simulink model "RaibertControlV13"  (R2022a)
settings: Solver=ode23t  StartTime=0.0  StopTime=10  FixedStep=1/1000  MaxStep=0.001  RelTol=1e-3  AbsTol=1e-3  EnableMultiTasking=on
values from neighbouring files (symbols this model uses):
  dphi_d_14 = 0.0    (= 0)    [initialization.m]
  dphi_d_23 = 0.0    (= 0)    [initialization.m]
  dphi_des = DesiredImpedenceValues(4)    [Controller.m]    (also in initialization.m = 0)
  dr_d_14 = 0.0    (= 0)    [initialization.m]
  dr_d_23 = 0.0    (= 0)    [initialization.m]
  dr_des = DesiredImpedenceValues(3)    [Controller.m]    (also in initialization.m = 0)
  Fpush_d_14 = 300    [initialization.m]
  Fpush_d_23 = 300    [initialization.m]
  GAIN_dx_d_14 = 0.05    [initialization.m]
  GAIN_dx_d_23 = 0.05    [initialization.m]
  join_legs = -1    [initialization.m]
  Kd_phi_d_14 = 10    [initialization.m]
  Kd_phi_d_23 = 10    [initialization.m]
  Kd_r_d_14 = Kp_r_d_14*0.1    (= 60)    [initialization.m]
  Kd_r_d_23 = Kp_r_d_23*0.1    (= 50)    [initialization.m]
  Kdphi_des = DesiredImpedenceValues(8)    [Controller.m]    (also in initialization.m = 5)
  Kdr_des = DesiredImpedenceValues(6)    [Controller.m]    (also in initialization.m = 700)
  Kp_phi_d_14 = 200    [initialization.m]
  Kp_phi_d_23 = 200    [initialization.m]
  Kp_r_d_14 = 600    [initialization.m]
  Kp_r_d_23 = 500    [initialization.m]
  Kpphi_des = DesiredImpedenceValues(7)    [Controller.m]    (also in initialization.m = 50)
  Kpr_des = DesiredImpedenceValues(5)    [Controller.m]    (also in initialization.m = 700)
  phi_d_14 = 0    [initialization.m]
  phi_d_23 = 0    [initialization.m]
  phi_des = DesiredImpedenceValues(2)    [Controller.m]    (also in initialization.m = 0)
  r_d_14 = 0.38    [initialization.m]
  r_d_23 = 0.38    [initialization.m]
  r_des = DesiredImpedenceValues(1)    [Controller.m]    (also in initialization.m = 0.4)
  rthrust_d_14 = 0.3    [initialization.m]
  rthrust_d_23 = 0.3    [initialization.m]
undefined symbols (not defined in the file or in its folder): Carrier, N, Ring, T, X, Y, Z
libraries: sm_lib x160, nesl_utility x25, Multibody_Parts_Lib x4, fl_lib x4
(part 1 of 8)
settings Model: Creator=user  LastModifiedBy=user
settings SolverCC: AutoScaleAbsTol=off  ZeroCrossAlgorithm=Adaptive  AutoInsertRateTranBlk=on  MaxZcPerStep=1
settings DataIOCC: LimitDataPoints=on  MaxDataPoints=10000
settings OptimizationCC: LifeSpan=inf
settings DebuggingCC: UnconnectedInputMsg=warning  UnconnectedOutputMsg=warning  UnconnectedLineMsg=warning  AllowSymbolicDim=off  SFUnexpectedBacktrackingDiag=warning  SFNoUnconditionalDefaultTransitionDiag=warning  SFExecutionAtInitializationDiag=none  SFMachineParentedDataDiag=warning  ArithmeticOperatorsInVariantConditions=warning
settings SFSimCC: SimUseLocalCustomCode=off  CustomCodeUndefinedFunction=UseInterfaceOnly
settings RTWCC: RTWUseLocalCustomCode=off  DLArmComputeVersion=19.05
settings CodeAppCC: StateflowObjectComments=on
settings GRTTargetCC: TargetLangStandard=C89/C90 (ANSI)
settings ConfigComp: CovMetricSettings=dw  CovSaveCumulativeToWorkspaceVar=on  CovSaveSingleToWorkspaceVar=on  CovExternalEMLEnable=off  CovSFcnEnable=off
settings SimscapeCC: SimscapeLogType=all  SimscapeLogSimulationStatistics=on  SimscapeLogDataHistory=10000
settings ExplorerConfigSet: InternalSimMechanicsExplorerSettings="<ExplorerConfiguration><canonicalview>planar_xy</canonicalview><AnimationSetting><BasePlaybackSpeed>1.0</BasePlaybackSpeed><PlaybackSpeedFactor>1.0</PlaybackSpeedFactor></AnimationSetting><TilePanel><TileInfo><Tiles Columns=\"1\" Count=\"1\" Rows=\"1\"><Column Weight=\"1\"/><Row Weight=\"1\"/><Tile Height=\"1\" Width=\"1\" X=\"0\" Y=\"0\"/></Tiles></TileInfo><SceneInfo><SceneViewer><BGColor><R>0.60000002384185791</R><G>0.60000002384185791</G><B>0.60000002384185791</B></BGColor><Camera><DoPerspective>off</DoPerspective><Position><X>-1.06238065184303165</X><Y>0.28591497324730003</Y><Z>-0.103858662281123768</Z></Position><Center><X>0.999999918886055106</X><Y>0.28591497324730003</Y><Z>-0.103858662281123768</Z></Center><Up><X>-0</X><Y>1</Y><Z>0</Z></Up><ViewLimDist>1</ViewLimDist><YLim>0.282634040177624779</YLim><XLim>0.661062811059710653</XLim></Camera></SceneViewer></SceneInfo></TilePanel><MechEditorPanel><Cameras/><GfxPanelCameraMap/><VideoCreator><PlaybackSpeedRatio>1.0</PlaybackSpeedRatio><FrameRate>30</FrameRate><VideoFormat>Motion JPEG AVI</VideoFormat><FrameSize>auto</FrameSize></VideoCreator></MechEditorPanel></ExplorerConfiguration>"

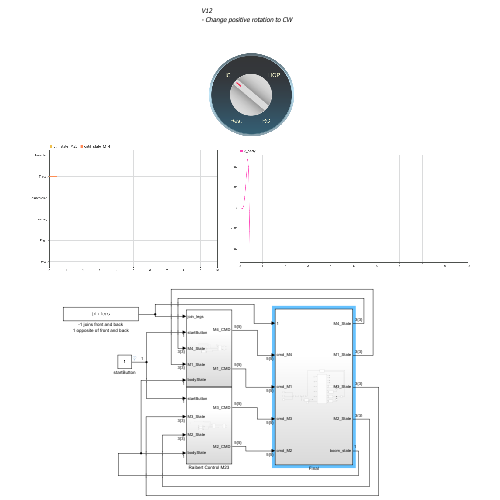
[thumbnail: Simulink's stored preview of the top-level diagram]
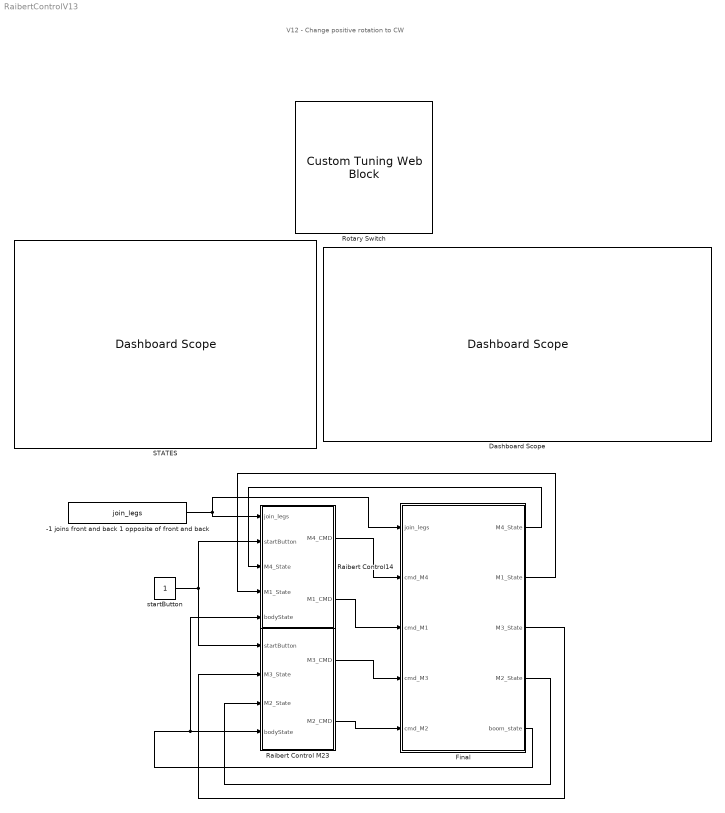
== system RaibertControlV13 ==
  note: V12
      | - Change positive rotation to CW
  -1 joins front and back 1 opposite of front and back : Constant  Value=join_legs
  Dashboard Scope : DashboardScope
  Final : Subsystem
  Raibert Control M23 : Subsystem
  Raibert Control14 : Subsystem
  Rotary Switch : CustomTuningWebBlock  LabelPosition=Hide  ShowInitialText=on  Configuration="{\"components\":[{\"name\":\"RotarySwitchComponent\",\"settings\":{\"arcAngle\":300,\"arcAngleOffset\":120,\"handle\":{\"size\":[150,150],\"src\":\"data:image\\/svg+xml;base64,PHN2ZyBpZD0iTGF5ZXJfMSIgZGF0YS1uYW1lPSJMYXllciAxIiB4bWxucz0iaHR0cDovL3d3dy53My5vcmcvMjAwMC9zdmciIHhtbG5zOnhsaW5rPSJodHRwOi8vd3d3LnczLm9yZy8xOTk5L3hsaW5rIiB2aWV3Qm94PSIwIDAgMTIxIDEyMSI+PGRlZnM+PHN0eWxlPi5jbHMtMXtmaWxsOnVybCgjbGluZWFyLWdyYWRpZW50KTt9LmNscy0yLC5jbHMtM3tmaWxsOiNkMWQxZDE7fS5jbHMtM3tzdHJva2U6I2I3YjdiNztzdHJva2UtbWl0ZXJsaW1pdDoxMDtzdHJva2Utd2lkdGg6MC4yNXB4O30uY2xzLTR7ZmlsbDojZjMwMDAwO30uY2xzLTV7ZmlsbDojZjIxNzY3O308L3N0eWxlPjxsaW5lYXJHcmFkaWVudCBpZD0ibGluZWFyLWdyYWRpZW50IiB4MT0iNjAuNSIgeTE9IjEyMC41IiB4Mj0iNjAuNSIgeTI9IjAuNSIgZ3JhZGllbnRVbml0cz0idXNlclNwYWNlT25Vc2UiPjxzdG9wIG9mZnNldD0iMCIgc3RvcC1jb2xvcj0iI2QxZDFkMSIvPjxzdG9wIG9mZnNldD0iMC4xIiBzdG9wLWNvbG9yPSIjY2VjZWNlIi8+PHN0b3Agb2Zmc2V0PSIwLjE5IiBzdG9wLWNvbG9yPSIjYzNjM2MzIi8+PHN0b3Agb2Zmc2V0PSIwLjI4IiBzdG9wLWNvbG9yPSIjYjFiMWIxIi8+PHN0b3Agb2Zmc2V0PSIwLjM2IiBzdG9wLWNvbG9yPSIjOTg5ODk4Ii8+PHN0b3Agb2Zmc2V0PSIwLjQ0IiBzdG9wLWNvbG9yPSIjNzg3ODc4Ii8+PHN0b3Agb2Zmc2V0PSIwLjQ2IiBzdG9wLWNvbG9yPSIjNmI2YjZiIi8+PHN0b3Agb2Zmc2V0PSIwLjU0IiBzdG9wLWNvbG9yPSIjNmI2YjZiIi8+PHN0b3Agb2Zmc2V0PSIwLjU2IiBzdG9wLWNvbG9yPSIjNzY3Njc2Ii8+PHN0b3Agb2Zmc2V0PSIwLjY0IiBzdG9wLWNvbG9yPSIjOTc5Nzk3Ii8+PHN0b3Agb2Zmc2V0PSIwLjcyIiBzdG9wLWNvbG9yPSIjYjBiMGIwIi8+PHN0b3Agb2Zmc2V0PSIwLjgxIiBzdG9wLWNvbG9yPSIjYzNjM2MzIi8+PHN0b3Agb2Zmc2V0PSIwLjkiIHN0b3AtY29sb3I9IiNjZGNkY2QiLz48c3RvcCBvZmZzZXQ9IjEiIHN0b3AtY29sb3I9IiNkMWQxZDEiLz48L2xpbmVhckdyYWRpZW50PjwvZGVmcz48Y2lyY2xlIGNsYXNzPSJjbHMtMSIgY3g9IjYwLjUiIGN5PSI2MC41IiByPSI2MCIvPjxwYXRoIGNsYXNzPSJjbHMtMiIgZD0iTTYwLjUsMUE1OS41LDU5LjUsMCwxLDEsMSw2MC41LDU5LjU3LDU5LjU3LDAsMCwxLDYwLjUsMW0wLTFBNjAuNSw2MC41LDAsMSwwLDEyMSw2MC41LDYwLjUsNjAuNSwwLDAsMCw2MC41LDBaIi8+PHJlY3QgY2xhc3M9ImNscy0zIiB4PSIwLjUiIHk9IjUxLjUiIHdpZHRoPSIxMjAiIGhlaWdodD0iMTgiIHJ4PSIzLjA0Ii8+PHJlY3QgY2xhc3M9ImNscy00IiB4PSI1Ljc1IiB5PSI1OC43NSIgd2lkdGg9IjE2IiBoZWlnaHQ9IjMiLz48cGF0aCBjbGFzcz0iY2xzLTUiIGQ9Ik0yMS4yNSw1OS4yNXYyaC0xNXYtMmgxNW0xLTFoLTE3djRoMTd2LTRaIi8+PC9zdmc+\"},\"handleOffset\":[0,0],\"handleOrientation\":180,\"handlePosition\":[0,0,1,1],\"handleSize\":{\"height\":0.5,\"width\":0.5},\"labelRadius\":0.36,\"position\":[0,0,1,1],\"states\":[{\"Label\":{\"color\":[0,0,0,1],\"icon\":{\"size\":[0,0],\"src\":[],\"srcOrientation\":\"Right\"},\"iconPlacement\":\"left\",\"opacity\":1,\"position\":[0.7345552884615385,0.6796274038461538],\"show\":true,\"text\":{\"content\":\"Rest\",\"font\":\"Helvetica\",\"fontSize\":24}},\"Value\":0},{\"Label\":{\"color\":[0,0,0,1],\"icon\":{\"size\":[0,0],\"src\":[],\"srcOrientation\":\"Right\"},\"iconPlacement\":\"left\",\"opacity\":1,\"position\":[0.35757211538461536,0.7603966346153846],\"show\":true,\"text\":{\"content\":\"IC\",\"font\":\"Helvetica\",\"fontSize\":24}},\"Value\":1},{\"Label\":{\"color\":[0,0,0,1],\"icon\":{\"size\":[0,0],\"src\":[],\"srcOrientation\":\"Right\"},\"iconPlacement\":\"left\",\"opacity\":1,\"position\":[0.09603365384615385,0.46033653846153844],\"show\":true,\"text\":{\"content\":\"HOP\",\"font\":\"Helvetica\",\"fontSize\":24}},\"Value\":2},{\"Label\":{\"color\":[0,0,0],\"icon\":{\"size\":[1,1],\"src\":\"default\",\"srcOrientation\":\"Right\"},\"iconPlacement\":\"left\",\"opacity\":1,\"position\":[0,0],\"show\":true,\"text\":{\"content\":\"RC\",\"fontSize\":14}},\"Value\":3}],\"tickRadius\":0.32}},{\"name\":\"BackgroundImageComponent\",\"settings\":{\"image\":{\"size\":[155,150],\"src\":\"data:image\\/svg+xml;base64,PD94bWwgdmVyc2lvbj0iMS4wIiBlbmNvZGluZz0idXRmLTgiPz4NCjwhLS0gR2VuZXJhdG9yOiBBZG9iZSBJbGx1c3RyYXRvciAyNS4wLjAsIFNWRyBFeHBvcnQgUGx1Zy1JbiAuIFNWRyBWZXJzaW9uOiA2LjAwIEJ1aWxkIDApICAtLT4NCjxzdmcgdmVyc2lvbj0iMS4xIg0KCSBpZD0iTGF5ZXJfMl8xXyIgeG1sbnM6Y2M9Imh0dHA6Ly9jcmVhdGl2ZWNvbW1vbnMub3JnL25zIyIgeG1sbnM6ZGM9Imh0dHA6Ly9wdXJsLm9yZy9kYy9lbGVtZW50cy8xLjEvIiB4bWxuczppbmtzY2FwZT0iaHR0cDovL3d3dy5pbmtzY2FwZS5vcmcv ...(+4184 chars)\",\"srcOrientation\":\"Right\"},\"position\":[0,0,1,1],\"scaleMode\":\"0\"}},{\"name\":\"ForegroundImageComponent\",\"settings\":{\"image\":{\"size\":[0,0],\"src\":\"default\",\"srcOrientation\":[]},\"isForeground\":1,\"position\":[0,0,1,1],\"scaleMode\":\"0\"}}],\"settings\":{\"BindingType\":\"param\",\"backgroundColor\":[0,0,255,\"1\"],\"enumDataType\":\"\",\"fixedAspectRatio\":\"off\",\"image\":{\"size\":[150,150],\"src\":\"data:image\\/svg+xml;base64,PD94bWwgdmVyc2lvbj0iMS4wIiBlbmNvZGluZz0iVVRGLTgiIHN0YW5kYWxvbmU9Im5vIj8+CjwhLS0gR2VuZXJhdG9yOiBBZG9iZSBJbGx1c3RyYXRvciAxOS4yLjEsIFNWRyBFeHBvcnQgUGx1Zy1JbiAuIFNWRyBWZXJzaW9uOiA2LjAwIEJ1aWxkIDApICAtLT4KCjxzdmcKICAgeG1sbnM6ZGM9Imh0dHA6Ly9wdXJsLm9yZy9kYy9lbGVtZW50cy8xLjEvIgogICB4bWxuczpjYz0iaHR0cDovL2NyZWF0aXZlY29tbW9ucy5vcmcvbnMjIgogICB4bWxuczpyZGY9Imh0dHA6Ly93d3cudzMub3JnLzE5OTkvMDIvMjItcmRmLXN5bnRh ...(+9660 chars)\"},\"showBackgroundColor\":false,\"useEnumDataType\":false,\"variant\":\"rotarySwitch\"},\"type\":\"RotarySwitch\"}"
  STATES : DashboardScope  Ymin=0  Ymax=6  NormalizeYAxis=on
  startButton : Constant
  wires:
  Raibert Control14/1(M4_CMD) -> Final/2(cmd_M4)
  Raibert Control14/2(M1_CMD) -> Final/3(cmd_M1)
  Raibert Control M23/2(M2_CMD) -> Final/5(cmd_M2)
  Final/4(M2_State) -> Raibert Control M23/3(M2_State)
  Final/2(M1_State) -> Raibert Control14/4(M1_State)
  Final/3(M3_State) -> Raibert Control M23/2(M3_State)
  Final/1(M4_State) -> Raibert Control14/3(M4_State)
  Raibert Control M23/1(M3_CMD) -> Final/4(cmd_M3)
  Final/5(boom_state) -> Raibert Control14/5(bodyState), Raibert Control M23/4(bodyState)
  startButton/1 -> Raibert Control14/2(startButton), Raibert Control M23/1(startButton)
  -1 joins front and back 1 opposite of front and back/1 -> Raibert Control14/1(join_legs), Final/1(join_legs)

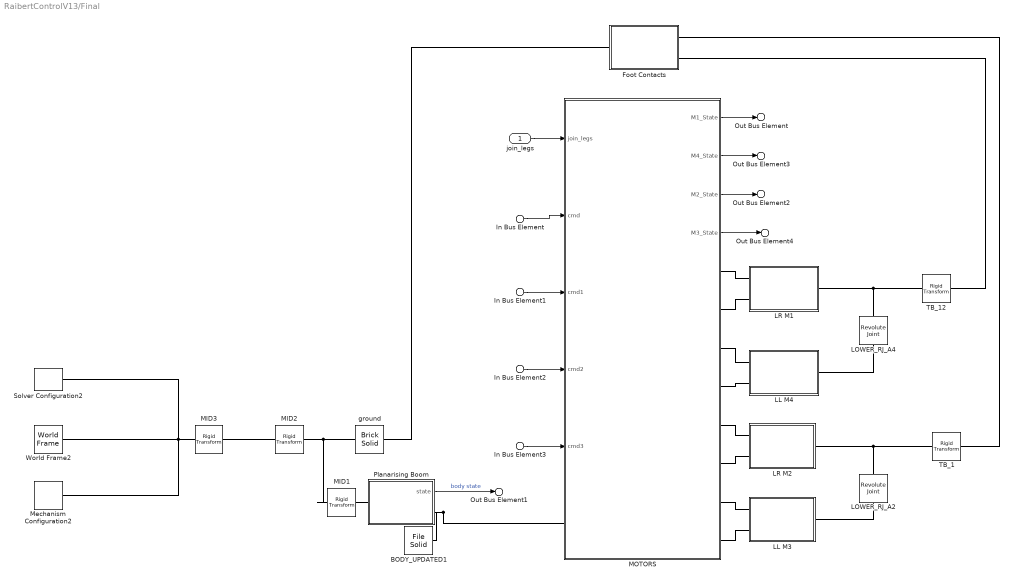
== system RaibertControlV13/Final ==
  join_legs : Inport
  In Bus Element1 : Inport  Port=2  PortName=cmd_M4
  In Bus Element : Inport  Port=3  PortName=cmd_M1
  In Bus Element3 : Inport  Port=4  PortName=cmd_M3
  In Bus Element2 : Inport  Port=5  PortName=cmd_M2
  BODY_UPDATED1 : sm_lib/Body Elements/File Solid  ExtGeomFileName=C:\Users\user\Desktop\Zubair\solidworks_simscape_setup\Rigid Bodies\updated\simscape files\Body.STL  UnitType=Custom  ExtGeomFileUnits=mm  StepReaderType=HEX  ExportConvexHullGeometry=off  InertiaType=Custom  Mass=5756.78  MassUnits=g  CenterOfMass=[0.00 8.34 76.00]  CenterOfMassUnits=mm  MomentsOfInertia="[19417888.32  38930926.54 32124078.52]"  MomentsOfInertiaUnits=g*mm^2  ProductsOfInertia=[0.00 522.32 0.00]  ProductsOfInertiaUnits=g*mm^2  BasedOnType=DensityFromFile  Density=1000  DensityUnits=kg/m^3  DoExposeReferenceFrame=on  SerializedFrames=<Frames/>  GraphicType=FromGeometry  MarkerShape=Sphere  MarkerSize=10  GraphicVisPropType=SimpleVisualProperties  GraphicDiffuseColor=[1.0 1.0 1.0]  GraphicSpecularColor=[0.5 0.5 0.5 1.0]  GraphicAmbientColor=[0.15 0.15 0.15 1.0]  GraphicEmissiveColor=[0.0 0.0 0.0 1.0]  GraphicShininess=75  GraphicOpacity=0.5
  Foot Contacts : Subsystem
  LL M3 : Subsystem
  LL M4 : Subsystem
  LOWER_RJ_A2 : sm_lib/Joints/Revolute Joint  JointMode=Normal  SenseConstraintForce=off  SenseConstraintForceX=off  SenseConstraintForceY=off  SenseConstraintForceZ=off  SenseConstraintTorque=off  SenseConstraintTorqueX=off  SenseConstraintTorqueY=off  SenseConstraintTorqueZ=off  SenseTotalForce=off  SenseTotalForceX=off  SenseTotalForceY=off  SenseTotalForceZ=off  SenseTotalTorque=off  SenseTotalTorqueX=off  SenseTotalTorqueY=off  SenseTotalTorqueZ=off  CompositeWrenchDir=FollowerOnBase  CompositeWrenchFrame=BaseFrame  EquilibriumPosition=0  EquilibriumPositionUnits=deg  SpringStiffness=0  SpringStiffnessUnits=N*m/deg  DampingCoefficient=0  DampingCoefficientUnits=N*m/(deg/s)  TorqueActuationMode=NoTorque  MotionActuationMode=ComputedMotion  SensePosition=off  SenseVelocity=off  SenseAcceleration=off  SenseTorqueForce=off  SenseLowerLimitTorqueForce=off  SenseUpperLimitTorqueForce=off  LowerLimitSpecify=off  LowerLimitBound=0  LowerLimitBoundUnits=deg  LowerLimitStiffness=1e4  LowerLimitStiffnessUnits=N*m/deg  LowerLimitDamping=10  LowerLimitDampingUnits=N*m/(deg/s)  LowerLimitTransitionRegionWidth=0.1  LowerLimitTransitionRegionWidthUnits=deg  UpperLimitSpecify=off  UpperLimitBound=0  UpperLimitBoundUnits=rad  UpperLimitStiffness=1e4  UpperLimitStiffnessUnits=N*m/deg  UpperLimitDamping=10  UpperLimitDampingUnits=N*m/(deg/s)  UpperLimitTransitionRegionWidth=0.1  UpperLimitTransitionRegionWidthUnits=deg  PositionTargetSpecify=off  PositionTargetPriority=High  PositionTargetValue=10  PositionTargetValueUnits=deg  VelocityTargetSpecify=off  VelocityTargetPriority=High  VelocityTargetValue=0  VelocityTargetValueUnits=deg/s
  LOWER_RJ_A4 : sm_lib/Joints/Revolute Joint  JointMode=Normal  SenseConstraintForce=off  SenseConstraintForceX=off  SenseConstraintForceY=off  SenseConstraintForceZ=off  SenseConstraintTorque=off  SenseConstraintTorqueX=off  SenseConstraintTorqueY=off  SenseConstraintTorqueZ=off  SenseTotalForce=off  SenseTotalForceX=off  SenseTotalForceY=off  SenseTotalForceZ=off  SenseTotalTorque=off  SenseTotalTorqueX=off  SenseTotalTorqueY=off  SenseTotalTorqueZ=off  CompositeWrenchDir=FollowerOnBase  CompositeWrenchFrame=BaseFrame  EquilibriumPosition=0  EquilibriumPositionUnits=deg  SpringStiffness=0  SpringStiffnessUnits=N*m/deg  DampingCoefficient=0  DampingCoefficientUnits=N*m/(deg/s)  TorqueActuationMode=NoTorque  MotionActuationMode=ComputedMotion  SensePosition=off  SenseVelocity=off  SenseAcceleration=off  SenseTorqueForce=off  SenseLowerLimitTorqueForce=off  SenseUpperLimitTorqueForce=off  LowerLimitSpecify=off  LowerLimitBound=0  LowerLimitBoundUnits=deg  LowerLimitStiffness=1e4  LowerLimitStiffnessUnits=N*m/deg  LowerLimitDamping=10  LowerLimitDampingUnits=N*m/(deg/s)  LowerLimitTransitionRegionWidth=0.1  LowerLimitTransitionRegionWidthUnits=deg  UpperLimitSpecify=off  UpperLimitBound=0  UpperLimitBoundUnits=deg  UpperLimitStiffness=1e4  UpperLimitStiffnessUnits=N*m/deg  UpperLimitDamping=10  UpperLimitDampingUnits=N*m/(deg/s)  UpperLimitTransitionRegionWidth=0.1  UpperLimitTransitionRegionWidthUnits=deg  PositionTargetSpecify=off  PositionTargetPriority=High  PositionTargetValue=10  PositionTargetValueUnits=deg  VelocityTargetSpecify=off  VelocityTargetPriority=High  VelocityTargetValue=0  VelocityTargetValueUnits=deg/s
  LR M1 : Subsystem
  LR M2 : Subsystem
  MID1 : sm_lib/Frames and Transforms/Rigid Transform  TranslationMethod=Cartesian  TranslationStandardOffset=700  TranslationLengthUnit=m  TranslationStandardAxis=-Y  TranslationCartesianOffset=[1 0 -0.1/2]  TranslationROffset=0  TranslationROffsetUnits=m  TranslationZOffset=0  TranslationZOffsetUnits=m  TranslationThetaOffset=0  TranslationThetaOffsetUnits=deg  RotationMethod=None  RotationAngleUnits=deg  RotationStandardAxis=+X  RotationAngle=90  RotationArbitraryAxis=[0 0 1]  FollAlignAxisA=+X  BaseAlignAxisA=+Y  FollAlignAxisB=+Y  BaseAlignAxisB=+Z  RotationSequenceAxes=FollowerAxes  RotationSequence=XYX  RotationSequenceAngles=[0 0 0]  RotationSequenceAnglesUnits=deg  RotationMatrix=[1 0 0; 0 1 0; 0 0 1]
  MID2 : sm_lib/Frames and Transforms/Rigid Transform  TranslationMethod=None  TranslationStandardOffset=1  TranslationLengthUnit=m  TranslationStandardAxis=-X  TranslationCartesianOffset=[0 0 0]  TranslationROffset=0  TranslationROffsetUnits=m  TranslationZOffset=0  TranslationZOffsetUnits=m  TranslationThetaOffset=0  TranslationThetaOffsetUnits=deg  RotationMethod=StandardAxis  RotationAngleUnits=deg  RotationStandardAxis=+Y  RotationAngle=180  RotationArbitraryAxis=[0 0 1]  FollAlignAxisA=+X  BaseAlignAxisA=+Y  FollAlignAxisB=+Y  BaseAlignAxisB=+Z  RotationSequenceAxes=FollowerAxes  RotationSequence=XYX  RotationSequenceAngles=[0 0 0]  RotationSequenceAnglesUnits=deg  RotationMatrix=[1 0 0; 0 1 0; 0 0 1]
  MID3 : sm_lib/Frames and Transforms/Rigid Transform  TranslationMethod=StandardAxis  TranslationStandardOffset=1  TranslationLengthUnit=m  TranslationStandardAxis=-X  TranslationCartesianOffset=[0 0 0]  TranslationROffset=0  TranslationROffsetUnits=m  TranslationZOffset=0  TranslationZOffsetUnits=m  TranslationThetaOffset=0  TranslationThetaOffsetUnits=deg  RotationMethod=StandardAxis  RotationAngleUnits=deg  RotationStandardAxis=+X  RotationAngle=-90  RotationArbitraryAxis=[0 0 1]  FollAlignAxisA=+X  BaseAlignAxisA=+Y  FollAlignAxisB=+Y  BaseAlignAxisB=+Z  RotationSequenceAxes=FollowerAxes  RotationSequence=XYX  RotationSequenceAngles=[0 0 0]  RotationSequenceAnglesUnits=deg  RotationMatrix=[1 0 0; 0 1 0; 0 0 1]
  MOTORS : Subsystem
  Mechanism Configuration2 : sm_lib/Utilities/Mechanism Configuration  UniformGravity=Constant  GravityVector=[0 -9.80665 0]  GravityUnits=m/s^2  LinearizationDelta=0.001  JointModeTransitionNonlinearIterations=2
  Planarising Boom : Subsystem
  Solver Configuration2 : nesl_utility/Solver Configuration  PhysicalDomain=network_engine_domain  SubClassName=solver  LeftPortType=input  RightPortType=generic  Tones=[]  Harmonics=[]  SimulateNoise=off  Profile=off  UseLocalSampling=off  EnableSwitchedLinearOptims=on  FrequencyDomain=off  UseCCode=off  RelTol=0.001  AbsTol=1e-06  MinStep=1e-09  ToWorkspace=off  RevertToSquareIcSolve=off  NumHomotopyIterations=100  PhasorMode=off  PhasorModeNumHarmonics=1  IndexReductionMethod=DerivativeReplacement  DoDC=off  ResidualTolerance=1e-09  UseLocalSolver=off  LocalSolverChoice=NE_BACKWARD_EULER_ADVANCER  LocalSolverSampleTime=0.001  DoFixedCost=off  MaxNonlinIter=3  MaxModeIter=2  ComputeImpulses=off  ImpulseIterations=2  LinearAlgebra=Sparse  LinearAlgebraNumThread=0  EquationFormulation=NE_TIME_EF  DelaysMemoryBudget=1024  AutomaticFiltering=on  FilteringTimeConstant=0.001  PartitionStorageMethod=AS_NEEDED  PartitionMemoryBudget=1024  PartitionMethod=FAST
      settings: SourceProductBaseCode=SS,PW,VE
  TB_1 : sm_lib/Frames and Transforms/Rigid Transform  TranslationMethod=Cartesian  TranslationStandardOffset=60  TranslationLengthUnit=mm  TranslationStandardAxis=-X  TranslationCartesianOffset=[-18.56 -18.56 0]  TranslationROffset=0  TranslationROffsetUnits=m  TranslationZOffset=0  TranslationZOffsetUnits=m  TranslationThetaOffset=0  TranslationThetaOffsetUnits=deg  RotationMethod=None  RotationAngleUnits=deg  RotationStandardAxis=+Z  RotationAngle=0.0  RotationArbitraryAxis=[0 0 1]  FollAlignAxisA=+Y  BaseAlignAxisA=+Y  FollAlignAxisB=+Z  BaseAlignAxisB=+X  RotationSequenceAxes=FollowerAxes  RotationSequence=XYX  RotationSequenceAngles=[0 0 0]  RotationSequenceAnglesUnits=deg  RotationMatrix=[1 0 0; 0 1 0; 0 0 1]
  TB_12 : sm_lib/Frames and Transforms/Rigid Transform  TranslationMethod=Cartesian  TranslationStandardOffset=60  TranslationLengthUnit=mm  TranslationStandardAxis=-X  TranslationCartesianOffset="[-18.56 -18.56  -18.56*0]"  TranslationROffset=0  TranslationROffsetUnits=m  TranslationZOffset=0  TranslationZOffsetUnits=m  TranslationThetaOffset=0  TranslationThetaOffsetUnits=deg  RotationMethod=None  RotationAngleUnits=deg  RotationStandardAxis=+Z  RotationAngle=0.0  RotationArbitraryAxis=[0 0 1]  FollAlignAxisA=+Y  BaseAlignAxisA=+Y  FollAlignAxisB=+Z  BaseAlignAxisB=+X  RotationSequenceAxes=FollowerAxes  RotationSequence=XYX  RotationSequenceAngles=[0 0 0]  RotationSequenceAnglesUnits=deg  RotationMatrix=[1 0 0; 0 1 0; 0 0 1]
  World Frame2 : sm_lib/Frames and Transforms/World Frame
  ground : sm_lib/Body Elements/Brick Solid  GraphicAmbientColor=[0.15 0.15 0.15 1.0]  BasedOnType=Density  BrickDimensions=[4 1 0.1]  BrickDimensionUnits=m  CenterOfMass=[0 0 0]  CenterOfMassUnits=m  GraphicDiffuseColor=[0.5 0.5 0.5]  Density=1000  DensityUnits=kg/m^3  DoExposeReferenceFrame=on  GraphicEmissiveColor=[0.0 0.0 0.0 1.0]  ExportEntireGeometry=on  SerializedFrames=<Frames/>  MarkerShape=Sphere  MarkerSize=10  GraphicType=FromGeometry  InertiaType=CalculateFromGeometry  Mass=1  MassUnits=kg  MomentsOfInertia=[1 1 1]  MomentsOfInertiaUnits=kg*m^2  GraphicOpacity=1.0  ProductsOfInertia=[0 0 0]  ProductsOfInertiaUnits=kg*m^2  GraphicShininess=75  GraphicSpecularColor=[0.5 0.5 0.5 1.0]  GraphicVisPropType=SimpleVisualProperties
  Out Bus Element3 : Outport  VectorParamsAs1DForOutWhenUnconnected=off  PortName=M4_State
  Out Bus Element : Outport  Port=2  VectorParamsAs1DForOutWhenUnconnected=off  PortName=M1_State
  Out Bus Element4 : Outport  Port=3  VectorParamsAs1DForOutWhenUnconnected=off  PortName=M3_State
  Out Bus Element2 : Outport  Port=4  VectorParamsAs1DForOutWhenUnconnected=off  PortName=M2_State
  Out Bus Element1 : Outport  Port=5  PortName=boom_state
  wires:
  Planarising Boom/1(state) -> Out Bus Element1/1  "body state"
  In Bus Element/1 -> MOTORS/2(cmd)
  In Bus Element1/1 -> MOTORS/3(cmd1)
  In Bus Element2/1 -> MOTORS/4(cmd2)
  In Bus Element3/1 -> MOTORS/5(cmd3)
  MOTORS/1(M1_State) -> Out Bus Element/1
  MOTORS/2(M4_State) -> Out Bus Element3/1
  MOTORS/3(M2_State) -> Out Bus Element2/1
  MOTORS/4(M3_State) -> Out Bus Element4/1
  join_legs/1 -> MOTORS/1(join_legs)
  connections:
  Planarising Boom/RConn1 -- BODY_UPDATED1/RConn1 -- MOTORS/LConn1
  ground/RConn1 -- MID1/RConn1 -- MID2/LConn1
  Planarising Boom/LConn1 -- MID1/LConn1
  LOWER_RJ_A2/LConn1 -- TB_1/LConn1 -- LR M2/RConn1
  MID3/RConn1 -- Mechanism Configuration2/RConn1 -- World Frame2/RConn1 -- Solver Configuration2/RConn1
  ground/LConn1 -- Foot Contacts/LConn1
  Foot Contacts/RConn2 -- TB_12/RConn1
  Foot Contacts/RConn1 -- TB_1/RConn1
  LR M1/RConn1 -- TB_12/LConn1 -- LOWER_RJ_A4/LConn1
  LR M1/LConn1 -- MOTORS/RConn1
  MOTORS/RConn3 -- LL M4/LConn1
  LOWER_RJ_A4/RConn1 -- LL M4/RConn1
  MOTORS/RConn5 -- LR M2/LConn1
  LL M3/LConn1 -- MOTORS/RConn7
  LL M3/RConn1 -- LOWER_RJ_A2/RConn1
  MID2/RConn1 -- MID3/LConn1
  LR M1/LConn2 -- MOTORS/RConn2
  MOTORS/RConn4 -- LL M4/LConn2
  LR M2/LConn2 -- MOTORS/RConn6
  LL M3/LConn2 -- MOTORS/RConn8

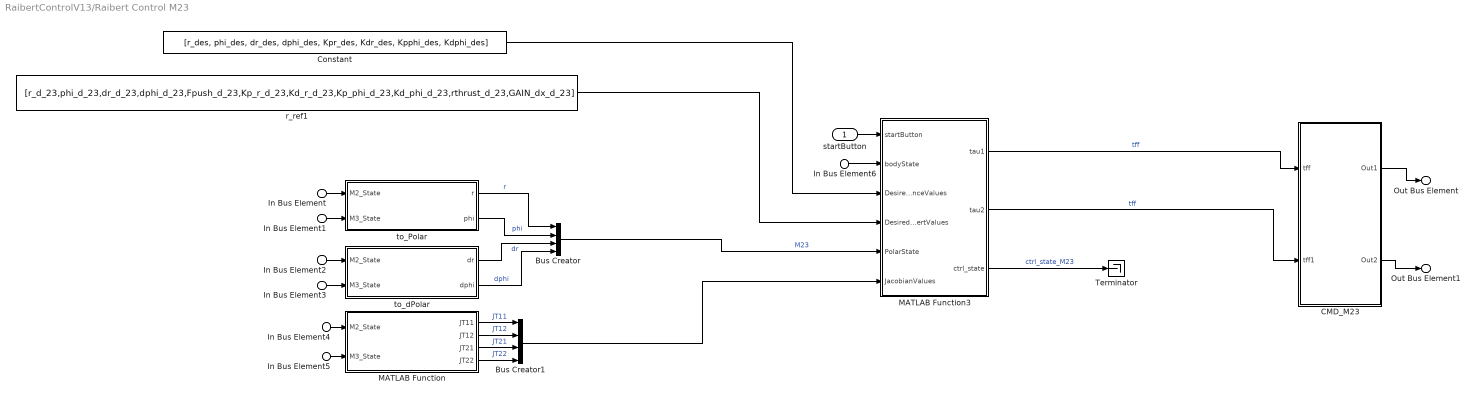
== system RaibertControlV13/Raibert Control M23 ==
  startButton : Inport
  In Bus Element1 : Inport  Port=2  PortName=M3_State
  In Bus Element3 : Inport  Port=2  PortName=M3_State
  In Bus Element5 : Inport  Port=2  PortName=M3_State
  In Bus Element : Inport  Port=3  PortName=M2_State
  In Bus Element2 : Inport  Port=3  PortName=M2_State
  In Bus Element4 : Inport  Port=3  PortName=M2_State
  In Bus Element6 : Inport  Port=4  PortName=bodyState
  Bus Creator : BusCreator  Inputs=4  OutDataTypeStr=Bus: PolarState
      settings: InheritFromInputs=off
  Bus Creator1 : BusCreator  Inputs=4  OutDataTypeStr=Bus: JacobianValues
  CMD_M23 : Subsystem
  Constant : Constant  Value=[r_des, phi_des, dr_des, dphi_des, Kpr_des, Kdr_des, Kpphi_des, Kdphi_des]
  MATLAB Function : MATLAB Function  TreatAsAtomicUnit=on
  MATLAB Function3 : MATLAB Function  TreatAsAtomicUnit=on
  Terminator : Terminator
  r_ref1 : Constant  Value=[r_d_23,phi_d_23,dr_d_23,dphi_d_23,Fpush_d_23,Kp_r_d_23,Kd_r_d_23,Kp_phi_d_23,Kd_phi_d_23,rthrust_d_23,GAIN_dx_d_23]
  to_Polar : MATLAB Function  TreatAsAtomicUnit=on
  to_dPolar : MATLAB Function  TreatAsAtomicUnit=on
  Out Bus Element : Outport  VectorParamsAs1DForOutWhenUnconnected=off  PortName=M3_CMD
  Out Bus Element1 : Outport  Port=2  VectorParamsAs1DForOutWhenUnconnected=off  PortName=M2_CMD
  wires:
  to_Polar/1(r) -> Bus Creator/1  "r"
  to_Polar/2(phi) -> Bus Creator/2  "phi"
  to_dPolar/1(dr) -> Bus Creator/3  "dr"
  to_dPolar/2(dphi) -> Bus Creator/4  "dphi"
  In Bus Element/1 -> to_Polar/1(M2_State)
  In Bus Element1/1 -> to_Polar/2(M3_State)
  In Bus Element2/1 -> to_dPolar/1(M2_State)
  In Bus Element3/1 -> to_dPolar/2(M3_State)
  MATLAB Function/1(JT11) -> Bus Creator1/1  "JT11"
  MATLAB Function/2(JT12) -> Bus Creator1/2  "JT12"
  MATLAB Function/3(JT21) -> Bus Creator1/3  "JT21"
  MATLAB Function/4(JT22) -> Bus Creator1/4  "JT22"
  Bus Creator1/1 -> MATLAB Function3/6(JacobianValues)
  In Bus Element4/1 -> MATLAB Function/1(M2_State)
  In Bus Element5/1 -> MATLAB Function/2(M3_State)
  Bus Creator/1 -> MATLAB Function3/5(PolarState)  "M23"
  In Bus Element6/1 -> MATLAB Function3/2(bodyState)
  MATLAB Function3/1(tau1) -> CMD_M23/1(tff)  "tff"
  MATLAB Function3/2(tau2) -> CMD_M23/2(tff1)  "tff"
  CMD_M23/1(Out1) -> Out Bus Element/1
  CMD_M23/2(Out2) -> Out Bus Element1/1
  startButton/1 -> MATLAB Function3/1(startButton)
  Constant/1 -> MATLAB Function3/3(DesiredImpedenceValues)
  r_ref1/1 -> MATLAB Function3/4(DesiredRaibertValues)
  MATLAB Function3/3(ctrl_state) -> Terminator/1  "ctrl_state_M23"

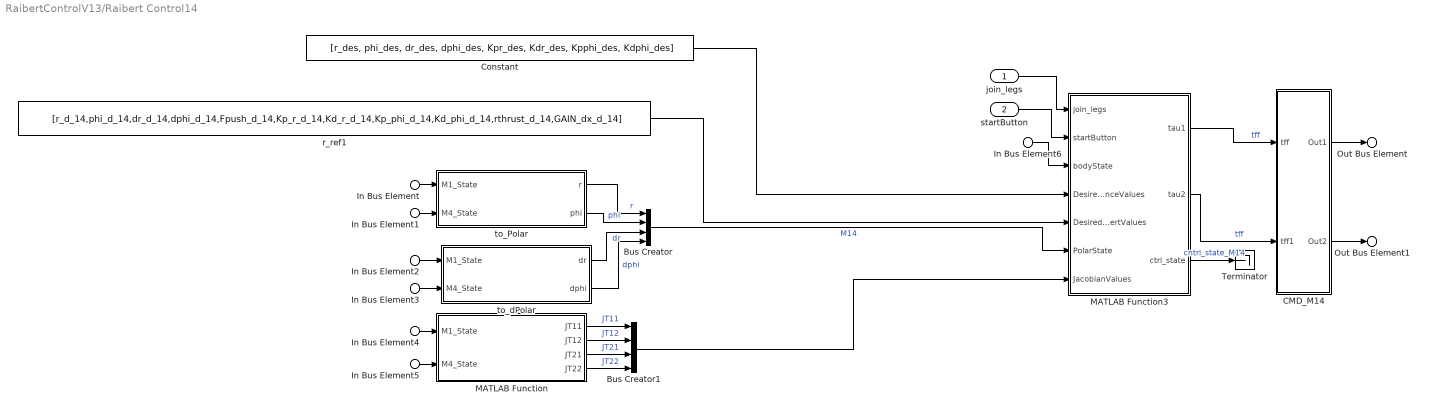
== system RaibertControlV13/Raibert Control14 ==
  join_legs : Inport
  startButton : Inport  Port=2
  In Bus Element1 : Inport  Port=3  PortName=M4_State
  In Bus Element3 : Inport  Port=3  PortName=M4_State
  In Bus Element5 : Inport  Port=3  PortName=M4_State
  In Bus Element : Inport  Port=4  PortName=M1_State
  In Bus Element2 : Inport  Port=4  PortName=M1_State
  In Bus Element4 : Inport  Port=4  PortName=M1_State
  In Bus Element6 : Inport  Port=5  PortName=bodyState
  Bus Creator : BusCreator  Inputs=4  OutDataTypeStr=Bus: PolarState
      settings: InheritFromInputs=off
  Bus Creator1 : BusCreator  Inputs=4  OutDataTypeStr=Bus: JacobianValues
  CMD_M14 : Subsystem
  Constant : Constant  Value=[r_des, phi_des, dr_des, dphi_des, Kpr_des, Kdr_des, Kpphi_des, Kdphi_des]
  MATLAB Function : MATLAB Function  TreatAsAtomicUnit=on
  MATLAB Function3 : MATLAB Function  TreatAsAtomicUnit=on
  Terminator : Terminator
  r_ref1 : Constant  Value=[r_d_14,phi_d_14,dr_d_14,dphi_d_14,Fpush_d_14,Kp_r_d_14,Kd_r_d_14,Kp_phi_d_14,Kd_phi_d_14,rthrust_d_14,GAIN_dx_d_14]
  to_Polar : MATLAB Function  TreatAsAtomicUnit=on
  to_dPolar : MATLAB Function  TreatAsAtomicUnit=on
  Out Bus Element : Outport  VectorParamsAs1DForOutWhenUnconnected=off  PortName=M4_CMD
  Out Bus Element1 : Outport  Port=2  VectorParamsAs1DForOutWhenUnconnected=off  PortName=M1_CMD
  wires:
  to_Polar/1(r) -> Bus Creator/1  "r"
  to_Polar/2(phi) -> Bus Creator/2  "phi"
  to_dPolar/1(dr) -> Bus Creator/3  "dr"
  to_dPolar/2(dphi) -> Bus Creator/4  "dphi"
  In Bus Element/1 -> to_Polar/1(M1_State)
  In Bus Element1/1 -> to_Polar/2(M4_State)
  In Bus Element2/1 -> to_dPolar/1(M1_State)
  In Bus Element3/1 -> to_dPolar/2(M4_State)
  MATLAB Function/1(JT11) -> Bus Creator1/1  "JT11"
  MATLAB Function/2(JT12) -> Bus Creator1/2  "JT12"
  MATLAB Function/3(JT21) -> Bus Creator1/3  "JT21"
  MATLAB Function/4(JT22) -> Bus Creator1/4  "JT22"
  Bus Creator1/1 -> MATLAB Function3/7(JacobianValues)
  In Bus Element4/1 -> MATLAB Function/1(M1_State)
  In Bus Element5/1 -> MATLAB Function/2(M4_State)
  Bus Creator/1 -> MATLAB Function3/6(PolarState)  "M14"
  In Bus Element6/1 -> MATLAB Function3/3(bodyState)
  MATLAB Function3/1(tau1) -> CMD_M14/1(tff)  "tff"
  MATLAB Function3/2(tau2) -> CMD_M14/2(tff1)  "tff"
  CMD_M14/1(Out1) -> Out Bus Element/1
  CMD_M14/2(Out2) -> Out Bus Element1/1
  startButton/1 -> MATLAB Function3/2(startButton)
  MATLAB Function3/3(ctrl_state) -> Terminator/1  "cntrl_state_M14"
  r_ref1/1 -> MATLAB Function3/5(DesiredRaibertValues)
  Constant/1 -> MATLAB Function3/4(DesiredImpedenceValues)
  join_legs/1 -> MATLAB Function3/1(join_legs)

== system RaibertControlV13/Final/Foot Contacts ==
  Cylindrical Solid1 : sm_lib/Body Elements/Cylindrical Solid  GraphicAmbientColor=[0.15 0.15 0.15 1.0]  BasedOnType=Density  CenterOfMass=[0 0 0]  CenterOfMassUnits=m  GraphicDiffuseColor=[0.5 0.5 0.5]  CylinderLength=35  CylinderLengthUnits=mm  CylinderRadius=16.25  CylinderRadiusUnits=mm  Density=1000  DensityUnits=kg/m^3  DoExposeReferenceFrame=on  GraphicEmissiveColor=[0.0 0.0 0.0 1.0]  ExportEntireGeometry=on  SerializedFrames=<Frames/>  MarkerShape=Sphere  MarkerSize=10  GraphicType=FromGeometry  InertiaType=Custom  Mass=0  MassUnits=kg  MomentsOfInertia=[0 0 0]  MomentsOfInertiaUnits=kg*m^2  GraphicOpacity=1.0  ProductsOfInertia=[0 0 0]  ProductsOfInertiaUnits=kg*m^2  GraphicShininess=75  GraphicSpecularColor=[0.5 0.5 0.5 1.0]  GraphicVisPropType=SimpleVisualProperties
  Cylindrical Solid2 : sm_lib/Body Elements/Cylindrical Solid  GraphicAmbientColor=[0.15 0.15 0.15 1.0]  BasedOnType=Density  CenterOfMass=[0 0 0]  CenterOfMassUnits=m  GraphicDiffuseColor=[0.5 0.5 0.5]  CylinderLength=35  CylinderLengthUnits=mm  CylinderRadius=16.25  CylinderRadiusUnits=mm  Density=1000  DensityUnits=kg/m^3  DoExposeReferenceFrame=on  GraphicEmissiveColor=[0.0 0.0 0.0 1.0]  ExportEntireGeometry=on  SerializedFrames=<Frames/>  MarkerShape=Sphere  MarkerSize=10  GraphicType=FromGeometry  InertiaType=Custom  Mass=0  MassUnits=kg  MomentsOfInertia=[0 0 0]  MomentsOfInertiaUnits=kg*m^2  GraphicOpacity=1.0  ProductsOfInertia=[0 0 0]  ProductsOfInertiaUnits=kg*m^2  GraphicShininess=75  GraphicSpecularColor=[0.5 0.5 0.5 1.0]  GraphicVisPropType=SimpleVisualProperties
  ORIGINAL : sm_lib/Forces and Torques/Spatial Contact Force  Commented=on  SenseContactBaseRotation=off  SenseContactBaseTranslation=off  CoefficientOfDynamicFriction=0.7  CoefficientOfStaticFriction=0.9  NormalDamping=1e3  NormalDampingUnits=N/(m/s)  SenseContactSignal=off  NormalStiffness=5e4  NormalStiffnessUnits=N/m  FrictionalCriticalVelocity=1e-3  FrictionalCriticalVelocityUnits=m/s  ZeroCrossDetectContactStartAndEnd=on  SenseContactFollowerRotation=off  SenseContactFollowerTranslation=off  FrictionType=SmoothStickSlip  SenseFrictionalForceMagnitude=off  SenseNormalForceMagnitude=off  NormalForceType=SmoothSpringDamper  SenseNormalVelocity=off  SenseSeparationDistance=off  SenseTangentialVelocity=off  NormalTransitionRegionWidth=1e-4  NormalTransitionRegionWidthUnits=m
  Spatial Contact Force : sm_lib/Forces and Torques/Spatial Contact Force  SenseContactBaseRotation=off  SenseContactBaseTranslation=off  CoefficientOfDynamicFriction=0.7  CoefficientOfStaticFriction=0.9  NormalDamping=1e4  NormalDampingUnits=N/(m/s)  SenseContactSignal=off  NormalStiffness=5e5  NormalStiffnessUnits=N/m  FrictionalCriticalVelocity=1e-3  FrictionalCriticalVelocityUnits=m/s  ZeroCrossDetectContactStartAndEnd=on  SenseContactFollowerRotation=off  SenseContactFollowerTranslation=off  FrictionType=SmoothStickSlip  SenseFrictionalForceMagnitude=off  SenseNormalForceMagnitude=off  NormalForceType=SmoothSpringDamper  SenseNormalVelocity=off  SenseSeparationDistance=off  SenseTangentialVelocity=off  NormalTransitionRegionWidth=1e-4  NormalTransitionRegionWidthUnits=m
  "Spatial Contact Force1  " : sm_lib/Forces and Torques/Spatial Contact Force  SenseContactBaseRotation=off  SenseContactBaseTranslation=off  CoefficientOfDynamicFriction=0.7  CoefficientOfStaticFriction=0.9  NormalDamping=1e4  NormalDampingUnits=N/(m/s)  SenseContactSignal=off  NormalStiffness=5e5  NormalStiffnessUnits=N/m  FrictionalCriticalVelocity=1e-3  FrictionalCriticalVelocityUnits=m/s  ZeroCrossDetectContactStartAndEnd=on  SenseContactFollowerRotation=off  SenseContactFollowerTranslation=off  FrictionType=SmoothStickSlip  SenseFrictionalForceMagnitude=off  SenseNormalForceMagnitude=off  NormalForceType=SmoothSpringDamper  SenseNormalVelocity=off  SenseSeparationDistance=off  SenseTangentialVelocity=off  NormalTransitionRegionWidth=1e-4  NormalTransitionRegionWidthUnits=m
  Ground : PMIOPort  Side=Left
  Foot23 : PMIOPort  Port=2  Side=Right
  Foot14 : PMIOPort  Port=3  Side=Right
  connections:
  "Spatial Contact Force1  "/LConn1 -- Ground/RConn1 -- Spatial Contact Force/LConn1
  Cylindrical Solid1/RConn1 -- Foot14/RConn1
  "Spatial Contact Force1  "/RConn1 -- Cylindrical Solid2/LConn1
  Spatial Contact Force/RConn1 -- Cylindrical Solid1/LConn1
  Cylindrical Solid2/RConn1 -- Foot23/RConn1
